simulink model "Udan_SOC"  (R2017b)
settings: Solver=FixedStepAuto  StartTime=0.0  StopTime=1000  FixedStep=0.1  RelTol=1e-3
values from neighbouring files (symbols this model uses):
  DenominatorOfIntegratorFactor = 100.0    [SOC_Stateflow.sldd]
  SOC_CalcSohLKT = 1.0    [SOC_Stateflow.sldd]
  SOC_CalcSOHTempLimit = 70.0    [SOC_Stateflow.sldd]
  SOC_CapPerCycle = 100.0    [SOC_Stateflow.sldd]
  SOC_CapTemp_HLimit = 200.0    [SOC_Stateflow.sldd]
  SOC_CapTemp_LLimit = 0.0    [SOC_Stateflow.sldd]
  Soc_ConfigInfo = 0    [SOC_Stateflow.sldd]
  SOC_DchgEndCalib = 0.0    [SOC_Stateflow.sldd]
  SOC_DiffVoltMin = 10.0    [SOC_Stateflow.sldd]
  SOC_DSOCJumpMax = 500.0    [SOC_Stateflow.sldd]
  SOC_EfficientHighLimit = 250.0    [SOC_Stateflow.sldd]
  SOC_EfficientLowLimit = 40.0    [SOC_Stateflow.sldd]
  SOC_EmptyAus = 0.0    [SOC_Stateflow.sldd]
  SOC_EnableOcv = 1.0    [SOC_Stateflow.sldd]
  SOC_END_CALIB_STATE : value not decoded    [SOC_Stateflow.sldd]
  SOC_HighRealSoc = 95.0    [SOC_Stateflow.sldd]
  SOC_LKTSohCycles = 0.0 1.0 10.0 20.0 30.0 40.0 50.0 60.0 70.0 80.0 90.0 100.0 110.0 120.0 130.0 140.0 150.0 160.0 170.0 180.0 190.0 200.0 210.0 220.0 230.0 240.0 250.0 260.0 270.0 280.0 290.0 300.0 310.0 320.0 330.0 340.0 350.0 360.0 370.0 380.0 390.0 400.0 410.0 420.0 430.0 440.0 450.0 460.0 470.0 480.0 490.0 500.0 510.0 520.0 530.0 540.0 550.0 560.0 570.0 580.0 590.0 600.0 610.0 620.0 630.0 640.0 650.0 660.0 670.0    [SOC_Stateflow.sldd]
  SOC_LKTSohTable = 1000.0 991.0 989.0 992.0 993.0 995.0 994.0 993.0 1000.0 997.0 1002.0 1000.0 992.0 1000.0 989.0 992.0 989.0 994.0 989.0 993.0 994.0 994.0 994.0 993.0 991.0 991.0 992.0 993.0 991.0 985.0 985.0 985.0 979.0 975.0 978.0 984.0 982.0 974.0 975.0 972.0 972.0 975.0 977.0 977.0 974.0 971.0 973.0 971.0 966.0 968.0 965.0 959.0 957.0 956.0 957.0 954.0 955.0 951.0 954.0 951.0 942.0 942.0 940.0 942.0 947.0 949.0    [SOC_Stateflow.sldd]
  SOC_LowRealSoc = 5.0    [SOC_Stateflow.sldd]
  SOC_NominalCap_AmS = 576000000.0    [SOC_Stateflow.sldd]
  SOC_NominalVol = 4000.0    [SOC_Stateflow.sldd]
  SOC_OCVTemp_HLimit = 106.0    [SOC_Stateflow.sldd]
  SOC_OCVTemp_LLimit = 29.0    [SOC_Stateflow.sldd]
  SOC_ShortCalibDSoc = 1.0    [SOC_Stateflow.sldd]
  SOC_SOCResolution = 10000.0    [SOC_Stateflow.sldd]
  SOC_SohCalcCapPercent = 8.0    [SOC_Stateflow.sldd]
  SOC_SohCalcHighLimit = 60.0    [SOC_Stateflow.sldd]
  SOC_SohCalcLowLimit = 10.0    [SOC_Stateflow.sldd]
  SOC_SohCalcMidLimit = 30.0    [SOC_Stateflow.sldd]
  SOC_SOHResolution = 1000.0    [SOC_Stateflow.sldd]
  SOC_State = <binary blob, 1163 chars, not shown>    [SOC_Stateflow.sldd]
  SOC_TempCap_CapBuffer : value not decoded    [SOC_Stateflow.sldd]
  SOC_TempCap_TempBuffer : value not decoded    [SOC_Stateflow.sldd]
  SocOcvCalib_ConfigInfo = 0.0    [SOC_Stateflow.sldd]
  SocOcvCalib_SocBuffer1 : value not decoded    [SOC_Stateflow.sldd]
  SocOcvCalib_TempBuffer : value not decoded    [SOC_Stateflow.sldd]
  SocOcvCalib_VoltageBuffer1 = 3300.0 3303.0 3305.0 3307.0 3310.0 3311.0 3313.0 3314.0 3316.0 3317.0 3319.0 3320.0 3322.0 3323.0 3325.0 3322.0 3323.0 3325.0 3310.0 3313.0 3315.0 3317.0 3320.0 3321.0 3323.0 3324.0 3326.0 3327.0 3329.0 3330.0 3332.0 3333.0 3335.0 3332.0 3333.0 3335.0 3320.0 3323.0 3325.0 3327.0 3330.0 3331.0 3333.0 3334.0 3336.0 3337.0 3339.0 3340.0 3342.0 3343.0 3345.0 3342.0 3343.0 3345.0 3330.0 3333.0 3335.0 3    [SOC_Stateflow.sldd]
  SOHCalibCycle = 10.0    [SOC_Stateflow.sldd]
undefined symbols (not defined in the file or in its folder): DatetimeM_GetReturnType, ParameterM_EeepParaIndexType, Soc_CumuLativeTypeType, SOC_EgthTempChgValue, Soc_EnergyBuffer, SOC_FithTempChgValue, SOC_FstSlowTempChgValue, SOC_FstTempChgValue, SOC_FthTempChgValue, SOC_MaxCap_AmS, SOC_SethTempChgValue, SOC_SixTempChgValue, SOC_SndSlowTempChgValue, SOC_SndTempChgValue, SOC_TrdSlowTempChgValue, SOC_TrdTempChgValue, SocDiagCalib_NoCalibReasonType
libraries: simulink x138, hdlsllib x24, dspindex x4
(part 10 of 10)

== matlab function Udan_SOC/SOC_Calculate/UdanSOCCalcn/CapAdder1/Enabled Subsystem1/Enabled Subsystem1/MATLAB Function ==
  data: u input; y output
function y = fcn(u)

y = uint8(1:1:length(u));

== matlab function Udan_SOC/SOC_Calculate/UdanSOCCalcn/Function-Call Subsystem4/MATLAB Function ==
  data: u input; y output
function y = fcn(u)

y = uint8(1:1:length(u));

== stateflow chart Udan_SOC/SOC_Calculate/UdanSOCCalcn/LKTSOC/Chart ==
  state triggerflag=CalcDiff(subtrahend,minuend,diff) [function]
    (default) -> (junction 50)
    (junction 50) -> (junction 51) [order 1] : [subtrahend<=minuend]{delta=minuend-subtrahend;}
    (junction 51) -> (junction 52) [order 1] : [delta>diff]
    (junction 50) -> (junction 53) [order 2] : {delta=subtrahend-minuend;}
    (junction 51) -> (junction 57) [order 2] : {out=0;}
    (junction 52) -> (junction 58) : {out=-1;}
    (junction 53) -> (junction 54) [order 1] : [delta>diff]
    (junction 53) -> (junction 55) [order 2] : {out=0;}
    (junction 54) -> (junction 56) : {out=1;}
    (junction 56) -> (junction 55)
    (junction 57) -> (junction 56)
    (junction 58) -> (junction 57)
    (junction 55) -> (junction 59) : {triggerflag=out;}
  (default) -> (junction 15) : % AdjustPackSOC
  (junction 15) -> (junction 16) [order 1] : [CalcDiff(PackSoc,RealSoc,DSocJumpMax)==1]
  (junction 15) -> (junction 17) [order 2]
  (junction 16) -> (junction 24) : {PackSocOut=RealSoc+DSocJumpMax;}
  (junction 17) -> (junction 18) [order 1] : [CalcDiff(PackSoc,RealSoc,DSocJumpMax)==-1]
  (junction 17) -> (junction 21) [order 2] : {PackSocOut=PackSoc;}
  (junction 18) -> (junction 23) : {PackSocOut=RealSoc-DSocJumpMax;}
  (junction 23) -> (junction 21)
  (junction 24) -> (junction 23)
  (junction 21) -> (junction 25)
  data: subtrahend function_input uint16; minuend function_input uint16; diff function_input int16; triggerflag function_output int8; delta local int16; out local int8; PackSoc input; RealSoc input; PackSocOut output uint16; DSocJumpMax input

== matlab function Udan_SOC/SOC_Calculate/UdanSOCCalcn/LKTSOC/MATLAB Function ==
  data: u input; y output
function y = fcn(u)

y = uint8(1:1:length(u));

== matlab function Udan_SOC/SOC_Calculate/UdanSOCCalcn/LKTSOC/MATLAB Function1 ==
  data: DeltaCap input; VoltBuffer input; LKTCap output; Index input; vol input
function LKTCap = fcn(DeltaCap,VoltBuffer,Index,vol)
minMaxTempVolt = uint16(VoltBuffer(15,1));
tmp = int32(0);
if vol < minMaxTempVolt
    LKTCap = int32(-DeltaCap+1);
else
    tmp = int32(DeltaCap)/int32((VoltBuffer(Index,1)-minMaxTempVolt));
    LKTCap = int32(-DeltaCap + tmp* int32((vol-minMaxTempVolt)));
end

== stateflow chart Udan_SOC/SOC_Calculate/UdanSOCCalcn/LKTSOC/Subsystem/Chart1 ==
  state triggerflag=CalcDiff(subtrahend,minuend,diff) [function]
    (default) -> (junction 15)
    (junction 15) -> (junction 16) [order 1] : [subtrahend<=minuend]{delta=minuend-subtrahend;}
    (junction 16) -> (junction 17) [order 1] : [delta>diff]
    (junction 15) -> (junction 18) [order 2] : {delta=subtrahend-minuend;}
    (junction 16) -> (junction 22) [order 2] : {out=0;}
    (junction 17) -> (junction 23) : {out=-1;}
    (junction 18) -> (junction 19) [order 1] : [delta>diff]
    (junction 18) -> (junction 20) [order 2] : {out=0;}
    (junction 19) -> (junction 21) : {out=1;}
    (junction 21) -> (junction 20)
    (junction 22) -> (junction 21)
    (junction 23) -> (junction 22)
    (junction 20) -> (junction 24) : {triggerflag=out;}
  (default) -> (junction 52)
  (junction 52) -> (junction 53) [order 1] : [CalcDiff(CalcSOH,EEEPSOH,MaxDiff)==0&&...
      | CalcDiff(CalcSOH,EEEPSOH,MaxCal1)!=0]
  (junction 53) -> (junction 63) [order 1] : [CalcDiff(CalcSOH,EEEPSOH,MaxCal)==0&&...
      | CalcDiff(CalcSOH,EEEPSOH,MaxCal1)!=0]
  (junction 63) -> (junction 89) [order 1] : [CalcDiff(CalcSOH,EEEPSOH,MaxCal1)==1]
  (junction 52) -> (junction 58) [order 2] : {SohOut=EEEPSOH;}
  (junction 53) -> (junction 67) [order 2]
  (junction 63) -> (junction 65) [order 2] : {SohOut=EEEPSOH-5;
      | SOHWriteResult=1;}
  (junction 89) -> (junction 91) : {SohOut=EEEPSOH+5;
      | SOHWriteResult=1;}
  (junction 67) -> (junction 68) [order 1] : [CalcDiff(CalcSOH,EEEPSOH,MaxCal)==-1]
  (junction 67) -> (junction 61) [order 2] : {SohOut=EEEPSOH+10;
      | SOHWriteResult=1;}
  (junction 68) -> (junction 70) : {SohOut=EEEPSOH-10;
      | SOHWriteResult=1;}
  (junction 61) -> (junction 58)
  (junction 70) -> (junction 61)
  (junction 65) -> (junction 70)
  (junction 91) -> (junction 65)
  (junction 58) -> (junction 62)
  data: subtrahend function_input uint16; minuend function_input uint16; diff function_input int16; triggerflag function_output int8; delta local int16; out local int8; CalcSOH input; SOHWriteResult output uint8; SohOut output uint16; MaxDiff input; MaxCal input; MaxCal1 input; EEEPSOH input
